simulink model "Boucle_de_regulation_P1"  (R2019b)
settings: Solver=ode1  StartTime=0.0  StopTime=1  FixedStep=Ts  RelTol=1e-3
values from neighbouring files (symbols this model uses):
  com = 1000    [Script_Propulseur_P1.m]
  f = 6.52e-6    (= 6.52e-06)    [Script_Propulseur_P1.m]
  gaincan = 2^10/3.3    (= 310.303030303)    [Script_Propulseur_P1.m]
  J = (Kem*Kem*tauEm)/Rm    (= 1.1664e-07)    [Script_Propulseur_P1.m]
  Kc = 1.602e-6    (= 1.602e-06)    [Script_Propulseur_P1.m]
  Kem = 2.7e-3    (= 0.0027)    [Script_Propulseur_P1.m]
  Kestvit = 1    [Script_Propulseur_P1.m]
  Lm = 2e-3    (= 0.002)    [Script_Propulseur_P1.m]
  pente = (8.2-6.9)/5    (= 0.26)    [Script_Propulseur_P1.m]
  Rm = 1    [Script_Propulseur_P1.m]
  tauf = Te*100    (= 0.005)    [Script_Propulseur_P1.m]
  Te = 5e-5    (= 5e-05)    [Script_Propulseur_P1.m]
  Ts = 0.5e-6    (= 5e-07)    [Script_Propulseur_P1.m]
libraries: simulink x3
settings Model: Creator=titil  LastModifiedBy=titil

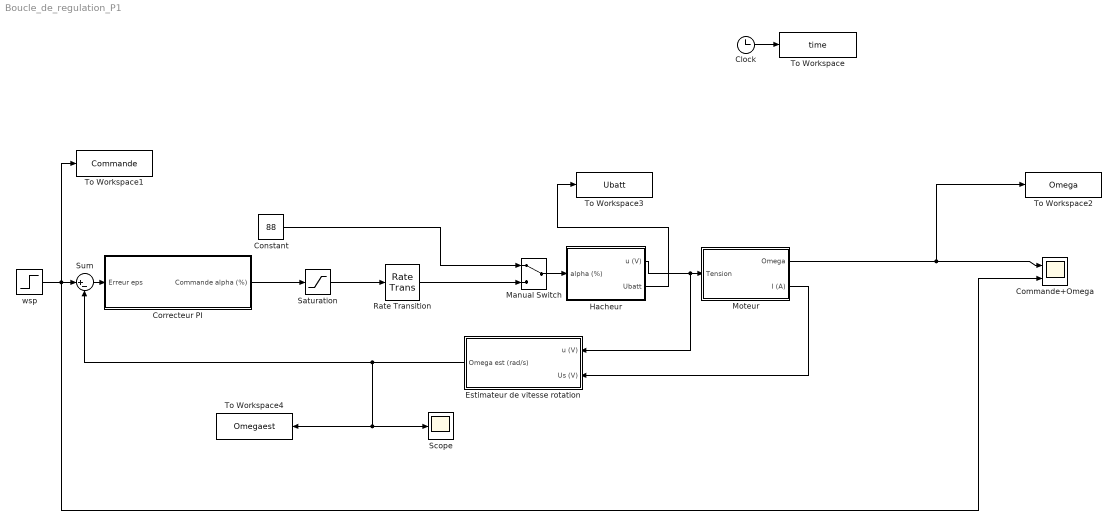
== system Boucle_de_regulation_P1 ==
  Clock : Clock
  Commande+Omega : Scope  NumInputPorts=2
  Constant : Constant  Value=88  SampleTime=Ts
  "Correcteur PI " : Subsystem
  Estimateur de vitesse rotation : Subsystem
  "Hacheur " : Subsystem
  Manual Switch : ManualSwitch
  Moteur : Subsystem
  Rate Transition : RateTransition  OutPortSampleTime=Ts
  Saturation : Saturate  UpperLimit=100  LowerLimit=0
  Scope : Scope
  Sum : Sum  Inputs=|+-
  To Workspace : ToWorkspace  VariableName=time  SampleTime=1e-3
      settings: Save2DSignal=2-D array (concatenate along first dimension)
  To Workspace1 : ToWorkspace  VariableName=Commande  SampleTime=1e-3
      settings: Save2DSignal=2-D array (concatenate along first dimension)
  To Workspace2 : ToWorkspace  VariableName=Omega  SampleTime=1e-3
      settings: Save2DSignal=2-D array (concatenate along first dimension)
  To Workspace3 : ToWorkspace  VariableName=Ubatt  SampleTime=1e-3
      settings: Save2DSignal=2-D array (concatenate along first dimension)
  To Workspace4 : ToWorkspace  VariableName=Omegaest  SampleTime=1e-3
      settings: Save2DSignal=2-D array (concatenate along first dimension)
  wsp : Step  Time=0  After=com  SampleTime=0
  wires:
  wsp/1 -> To Workspace1/1, Commande+Omega/2, Sum/1
  "Hacheur "/1(u (V)) -> Estimateur de vitesse rotation/1(u (V)), Moteur/1(Tension)
  Moteur/2(I (A)) -> Estimateur de vitesse rotation/2(Us (V))
  Manual Switch/1 -> "Hacheur "/1(alpha (%))
  Constant/1 -> Manual Switch/1
  Sum/1 -> "Correcteur PI "/1(Erreur eps)
  "Correcteur PI "/1(Commande alpha (%)) -> Saturation/1
  Moteur/1(Omega) -> To Workspace2/1, Commande+Omega/1
  Saturation/1 -> Rate Transition/1
  Rate Transition/1 -> Manual Switch/2
  Estimateur de vitesse rotation/1(Omega est (rad/s)) -> To Workspace4/1, Scope/1, Sum/2
  Clock/1 -> To Workspace/1
  "Hacheur "/2(Ubatt) -> To Workspace3/1

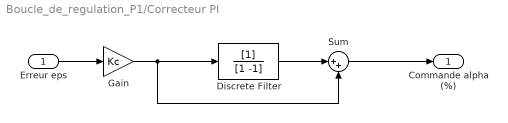
== system Boucle_de_regulation_P1/Correcteur PI  ==
  Erreur eps : Inport
  Discrete Filter : DiscreteFilter  Denominator=[1 -1]  SampleTime=Ts
  Gain : Gain  Gain=Kc
  Sum : Sum  Inputs=|++
  Commande alpha (%) : Outport
  wires:
  Erreur eps/1 -> Gain/1
  Gain/1 -> Sum/2, Discrete Filter/1
  Discrete Filter/1 -> Sum/1
  Sum/1 -> Commande alpha (%)/1

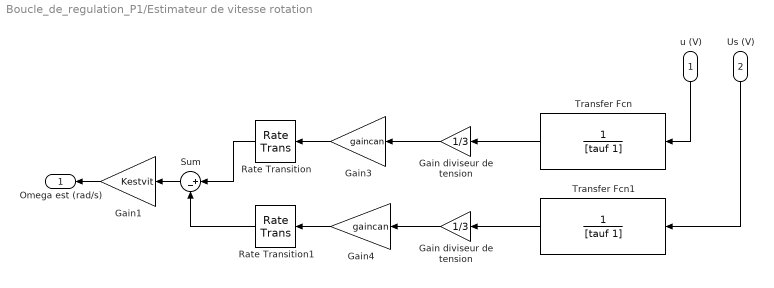
== system Boucle_de_regulation_P1/Estimateur de vitesse rotation ==
  u (V) : Inport
  Us (V) : Inport  Port=2
  Gain diviseur de tension : Gain  Gain=1/3
  "Gain diviseur de tension " : Gain  Gain=1/3
  Gain1 : Gain  Gain=Kestvit
  Gain3 : Gain  Gain=gaincan
  Gain4 : Gain  Gain=gaincan
  Rate Transition : RateTransition  OutPortSampleTime=1e-3
  Rate Transition1 : RateTransition  OutPortSampleTime=1e-3
  Sum : Sum  Inputs=|+-
  Transfer Fcn : TransferFcn  Denominator=[tauf 1]
  Transfer Fcn1 : TransferFcn  Denominator=[tauf 1]
  Omega est (rad/s) : Outport
  wires:
  Transfer Fcn/1 -> "Gain diviseur de tension "/1
  u (V)/1 -> Transfer Fcn/1
  Us (V)/1 -> Transfer Fcn1/1
  Transfer Fcn1/1 -> Gain diviseur de tension/1
  "Gain diviseur de tension "/1 -> Gain3/1
  Gain diviseur de tension/1 -> Gain4/1
  Gain1/1 -> Omega est (rad/s)/1
  Sum/1 -> Gain1/1
  Gain3/1 -> Rate Transition/1
  Rate Transition/1 -> Sum/1
  Gain4/1 -> Rate Transition1/1
  Rate Transition1/1 -> Sum/2

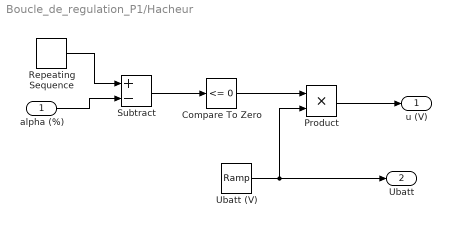
== system Boucle_de_regulation_P1/Hacheur  ==
  alpha (%) : Inport
  Compare To Zero : simulink/Logic and Bit Operations/Compare To Zero  relop=<=  OutDataTypeStr=boolean
  Product : Product
  Repeating Sequence : simulink/Sources/Repeating Sequence  rep_seq_t=[0 Te]  rep_seq_y=[1 100]
  Subtract : Sum  Inputs=+-
  Ubatt (V) : simulink/Sources/Ramp  slope=-pente  start=0  InitialOutput=8.2
  u (V) : Outport
  Ubatt : Outport  Port=2
  wires:
  Subtract/1 -> Compare To Zero/1
  Ubatt (V)/1 -> Ubatt/1, Product/2
  Product/1 -> u (V)/1
  Compare To Zero/1 -> Product/1
  Repeating Sequence/1 -> Subtract/1
  alpha (%)/1 -> Subtract/2

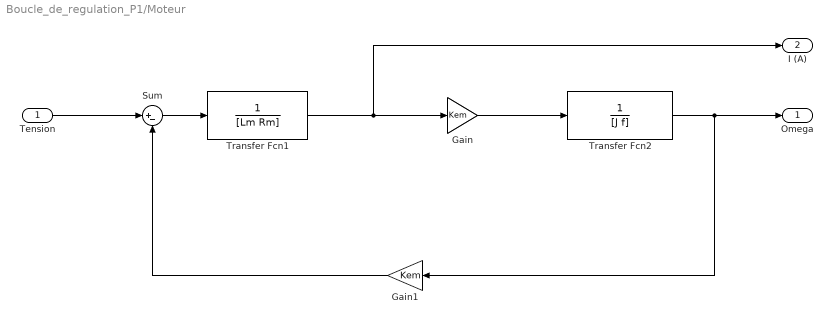
== system Boucle_de_regulation_P1/Moteur ==
  Tension : Inport
  Gain : Gain  Gain=Kem
  Gain1 : Gain  Gain=Kem
  Sum : Sum  Inputs=|+-
  Transfer Fcn1 : TransferFcn  Denominator=[Lm Rm]
  Transfer Fcn2 : TransferFcn  Denominator=[J f]
  Omega : Outport
  I (A) : Outport  Port=2
  wires:
  Sum/1 -> Transfer Fcn1/1
  Gain1/1 -> Sum/2
  Transfer Fcn2/1 -> Omega/1, Gain1/1
  Transfer Fcn1/1 -> I (A)/1, Gain/1
  Gain/1 -> Transfer Fcn2/1
  Tension/1 -> Sum/1
